simulink model "fixedwing_dynamics"  (R2024a)
settings: Solver=VariableStepAuto  StartTime=0.0  StopTime=10.0  RelTol=1e-3
undefined symbols (not defined in the file): I_xx, I_yy, I_zz, p, phi, psi, q, r, theta, v, w
libraries: aerolibobsolete x1, aerolibasang x1
settings Model: Creator=nikhi  LastModifiedBy=nikhi

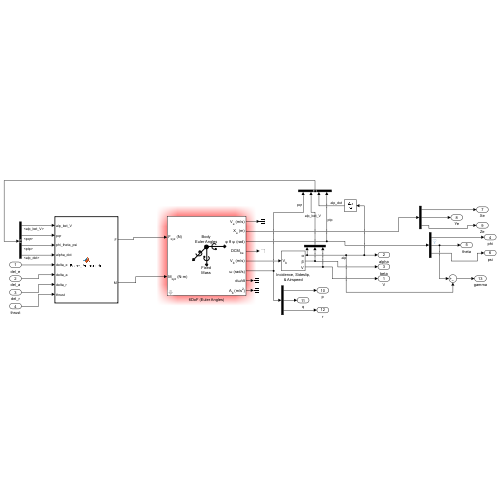
[thumbnail: Simulink's stored preview of the top-level diagram]
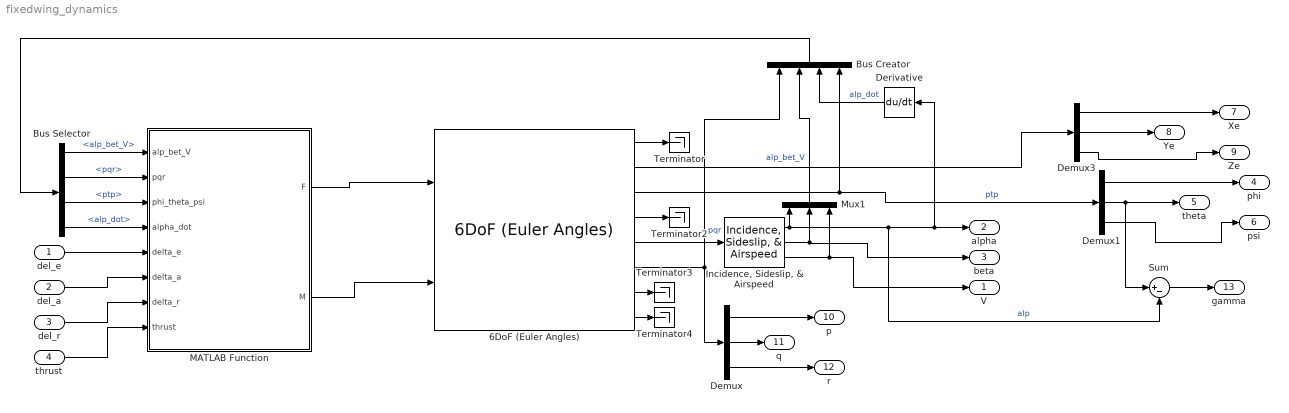
== system fixedwing_dynamics ==
  del_e : Inport
  del_a : Inport  Port=2
  del_r : Inport  Port=3
  thrust : Inport  Port=4
  6DoF (Euler Angles) : aerolibobsolete/6DoF (Euler Angles)  units=Metric (MKS)  mtype=Fixed  rep=Euler Angles  xme_0=[0 0 0]  Vm_0=[u v w]  eul_0=[phi theta psi]  pm_0=[p q r]  mass_0=m  mass_e=0.5  mass_f=2.0  inertia=diag([I_xx I_yy I_zz])  inertia_e=eye(3)  inertia_f=2*eye(3)  k_quat=1.0
  Bus Creator : BusCreator  Inputs=4
  Bus Selector : BusSelector  OutputSignals=alp_bet_V,pqr,ptp,alp_dot
  Demux : Demux  Outputs=3
  Demux1 : Demux  Outputs=3
  Demux3 : Demux  Outputs=3
  Derivative : Derivative
  "Incidence, Sideslip, & Airspeed" : aerolibasang/Incidence, Sideslip, & Airspeed
  MATLAB Function : MATLAB Function  TreatAsAtomicUnit=on
  Mux1 : Mux  Inputs=3
  Sum : Sum  Inputs=|+-
  Terminator{,2..4} (4 alike) : Terminator
  V : Outport
  alpha : Outport  Port=2
  beta : Outport  Port=3
  phi : Outport  Port=4
  theta : Outport  Port=5
  psi : Outport  Port=6
  Xe : Outport  Port=7
  Ye : Outport  Port=8
  Ze : Outport  Port=9
  p : Outport  Port=10
  q : Outport  Port=11
  r : Outport  Port=12
  gamma : Outport  Port=13
  wires:
  6DoF (Euler Angles)/3 -> Bus Creator/4, Demux1/1  "ptp"
  MATLAB Function/2(M) -> 6DoF (Euler Angles)/2
  Demux3/1 -> Xe/1
  Sum/1 -> gamma/1
  Demux1/3 -> psi/1
  del_r/1 -> MATLAB Function/7(delta_r)
  "Incidence, Sideslip, & Airspeed"/3 -> V/1, Mux1/3
  6DoF (Euler Angles)/4 -> Terminator2/1
  Bus Selector/4 -> MATLAB Function/4(alpha_dot)  "<alp_dot>"
  6DoF (Euler Angles)/7 -> Terminator3/1
  Demux/3 -> r/1
  thrust/1 -> MATLAB Function/8(thrust)
  Bus Selector/3 -> MATLAB Function/3(phi_theta_psi)  "<ptp>"
  del_a/1 -> MATLAB Function/6(delta_a)
  Demux3/3 -> Ze/1
  6DoF (Euler Angles)/8 -> Terminator4/1
  Derivative/1 -> Bus Creator/3  "alp_dot"
  Demux3/2 -> Ye/1
  Demux/1 -> p/1
  6DoF (Euler Angles)/2 -> Demux3/1
  6DoF (Euler Angles)/5 -> "Incidence, Sideslip, & Airspeed"/1
  del_e/1 -> MATLAB Function/5(delta_e)
  6DoF (Euler Angles)/1 -> Terminator/1
  "Incidence, Sideslip, & Airspeed"/1 -> alpha/1, Derivative/1, Sum/2, Mux1/1  "alp"
  MATLAB Function/1(F) -> 6DoF (Euler Angles)/1
  Demux1/2 -> theta/1, Sum/1
  Bus Selector/1 -> MATLAB Function/1(alp_bet_V)  "<alp_bet_V>"
  Bus Selector/2 -> MATLAB Function/2(pqr)  "<pqr>"
  Bus Creator/1 -> Bus Selector/1
  6DoF (Euler Angles)/6 -> Bus Creator/1, Demux/1  "pqr"
  Demux/2 -> q/1
  Mux1/1 -> Bus Creator/2  "alp_bet_V"
  Demux1/1 -> phi/1
  "Incidence, Sideslip, & Airspeed"/2 -> beta/1, Mux1/2

== matlab function fixedwing_dynamics/MATLAB Function ==
  data: alp_bet_V input; F output; pqr input; phi_theta_psi input; M output; alpha_dot input; delta_e input; delta_a input; delta_r input; thrust input
function [F, M] = Force_Aerosonde(alp_bet_V, pqr, phi_theta_psi, alpha_dot, delta_e, delta_a, delta_r, thrust)
F = zeros([3 1]);
M = zeros([3 1]);

alpha = alp_bet_V(1);
beta = alp_bet_V(2);
V = alp_bet_V(3);

p = pqr(1);
q = pqr(2);
r = pqr(3);

phi = phi_theta_psi(1);
theta = phi_theta_psi(2);
psi = phi_theta_psi(3);

g = 9.8;
rho = 1.2682;

m = 17;     % 1)a)11.458, b)+1.9344, c)+2.1625
C_bar = 0.18994;                    
b = 2.8956;
S_ref = 0.55;

C_L_0 = 0.28;
C_L_alpha = 3.45;
C_L_q = 0;
C_L_delta_e = -0.36;

% Ignore all other C_D derivatives excluding C_D_0
% Use C_D = C_D_0 + k*C_L^2

C_D_0 = 0.03 + 0.0172724;            % C_D_p (Using formula in book)
k = 0.023199;                       % 1/pi*e*AR

C_Y_beta = -0.98;
C_Y_p = 0;
C_Y_r = 0;
C_Y_delta_a = 0;
C_Y_delta_r = -0.17;                 % Added the parameter 

C_l_beta = -0.12;
C_l_p = -0.26;
C_l_r = 0.14;
C_l_delta_a = 0.08;
C_l_delta_r = 0.105;

C_M_0 = -0.02338;
C_M_alpha = -0.38;
C_M_alpha_dot = 0;              
C_M_q = -3.6;                   % Added the parameter
C_M_delta_e = -0.5;

C_N_beta = 0.25;
C_N_p = 0.022;
C_N_r = -0.35;
C_N_delta_a = 0.06;
C_N_delta_r = -0.032;


% CL using a Blending function "sigma"
M_sigma       = 50; 
alpha_0 = 0.4712;

CL_wing = C_L_0 + C_L_alpha*alpha + C_L_q*(q*C_bar/(2*V)) + C_L_delta_e*delta_e;

% Plate lift coefficient (already symmetric for alpha)
CL_plate = 2 * sign(alpha) * sin(alpha)^2 * cos(alpha);

% Blending function for symmetry
sigma   = (1 + exp(-M_sigma*(alpha-alpha_0)) + exp(M_sigma*(alpha+alpha_0)))/...
          ((1 + exp(-M_sigma*(alpha-alpha_0)))*(1 + exp(M_sigma*(alpha+alpha_0))));








C_L = (1 - sigma) * CL_wing + sigma * CL_plate;
C_D = C_D_0 + k*C_L^2;
C_Y = C_Y_beta*beta + C_Y_p*(p*b/(2*V)) + C_Y_r*(r*b/(2*V)) + C_Y_delta_a*delta_a + C_Y_delta_r*delta_r;

C_l = C_l_beta*beta + C_l_p*(p*b/(2*V)) + C_l_r*(r*b/(2*V)) + C_l_delta_a*delta_a + C_l_delta_r*delta_r;
C_M = C_M_0 + C_M_alpha*alpha + C_M_alpha_dot*(alpha_dot*C_bar/(2*V)) + C_M_delta_e*delta_e + C_M_q*(q*C_bar/(2*V));
C_N = C_N_beta*beta + C_N_p*(p*b/(2*V)) + C_N_r*(r*b/(2*V)) + C_N_delta_a*delta_a + C_N_delta_r*delta_r;

C_X = -C_D*cos(alpha) + C_L*sin(alpha);
C_Z = -C_D*sin(alpha) - C_L*cos(alpha);

F = zeros(3,1);
M = zeros(3,1);

q_bar = 0.5*rho*V*V;

F(1,1) = q_bar*S_ref*C_X - m*g*sin(theta) + thrust;
F(2,1) = q_bar*S_ref*C_Y + m*g*cos(theta)*sin(phi);
F(3,1) = q_bar*S_ref*C_Z + m*g*cos(theta)*cos(phi);

M(1,1) = q_bar*b*S_ref*C_l;
M(2,1) = q_bar*C_bar*S_ref*C_M;
M(3,1) = q_bar*b*S_ref*C_N;
